simulink model "fm_radio_simulink_v1"  (R2025b)
settings: Solver=VariableStepAuto  StartTime=0.0  StopTime=SimTime  RelTol=1e-3
undefined symbols (not defined in the file): a_de, b_de, decim1, decim2, decim3, decim4, fs_rf
libraries: dspmlti4 x4, dspsrcs4 x1
settings Model: SimulationMode=accelerator  Creator=kmuws  LastModifiedBy=kmuws

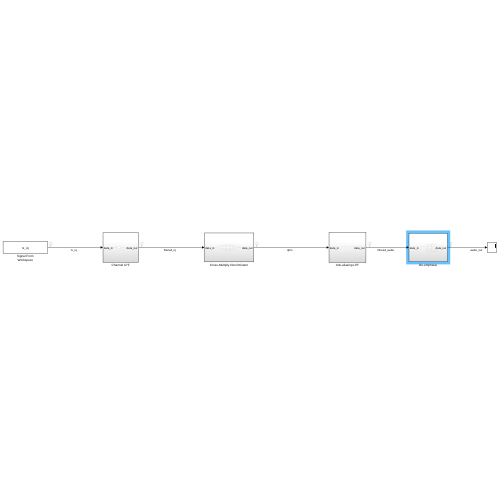
[thumbnail: Simulink's stored preview of the top-level diagram]
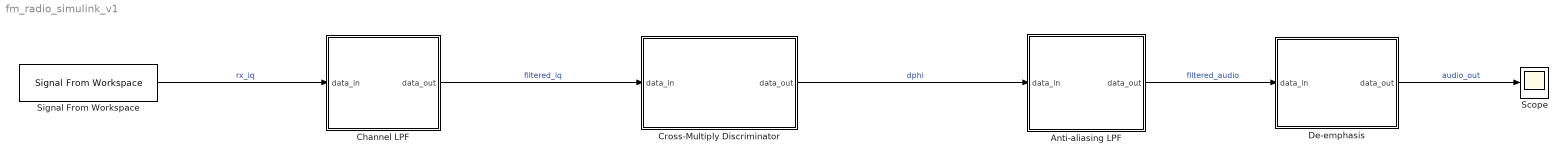
== system fm_radio_simulink_v1 ==
  Anti-aliasing LPF : Subsystem
  Channel LPF : Subsystem
  Cross-Multiply Discriminator : Subsystem
  De-emphasis : Subsystem
  Scope : Scope
      settings: ActiveDisplayYMinimum=-4.7153159237357389  ActiveDisplayYMaximum=3.7645676239050516
  Signal From Workspace : dspsrcs4/Signal From Workspace  X=rx_iq  Ts=1/fs_rf  nsamps=1  OutputAfterFinalValue=Setting to zero  ignoreOrWarnInputAndFrameLengths=off  OutputFrames=off
  wires:
  Signal From Workspace/1 -> Channel LPF/1(data_in)  "rx_iq"
  Channel LPF/1(data_out) -> Cross-Multiply Discriminator/1(data_in)  "filtered_iq"
  Cross-Multiply Discriminator/1(data_out) -> Anti-aliasing LPF/1(data_in)  "dphi"
  Anti-aliasing LPF/1(data_out) -> De-emphasis/1(data_in)  "filtered_audio"
  De-emphasis/1(data_out) -> Scope/1  "audio_out"

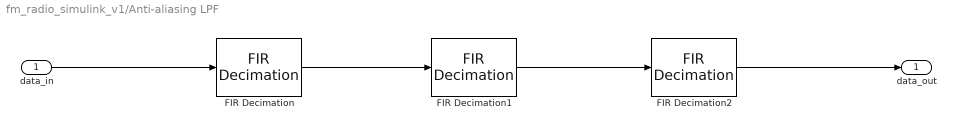
== system fm_radio_simulink_v1/Anti-aliasing LPF ==
  data_in : Inport
  FIR Decimation : dspmlti4/FIR Decimation  FilterSource=Dialog parameters  h=CoefFilter2  D=decim2  filtStruct=Direct form  FilterObject=FDECIM  framing=Enforce single-rate processing  AllowArbitraryInputLength=off  inputOffset=0  outputBufInitCond=0  roundingMode=Floor  overflowMode=off  firstCoeffDataTypeStr=Inherit: Same word length as input  firstCoeffMin=[]  firstCoeffMax=[]  firstCoeffLastDataTypeStr=Inherit: Same word length as input  outputDataTypeStr=Inherit: Same as accumulator  outputMin=[]  outputMax=[]  outputLastDataTypeStr=Inherit: Same as accumulator
  FIR Decimation1 : dspmlti4/FIR Decimation  FilterSource=Dialog parameters  h=CoefFilter3  D=decim3  filtStruct=Direct form  FilterObject=FDECIM  framing=Enforce single-rate processing  AllowArbitraryInputLength=off  inputOffset=0  outputBufInitCond=0  roundingMode=Floor  overflowMode=off  firstCoeffDataTypeStr=Inherit: Same word length as input  firstCoeffMin=[]  firstCoeffMax=[]  firstCoeffLastDataTypeStr=Inherit: Same word length as input  outputDataTypeStr=Inherit: Same as accumulator  outputMin=[]  outputMax=[]  outputLastDataTypeStr=Inherit: Same as accumulator
  FIR Decimation2 : dspmlti4/FIR Decimation  FilterSource=Dialog parameters  h=CoefFilter4  D=decim4  filtStruct=Direct form  FilterObject=FDECIM  framing=Enforce single-rate processing  AllowArbitraryInputLength=off  inputOffset=0  outputBufInitCond=0  roundingMode=Floor  overflowMode=off  firstCoeffDataTypeStr=Inherit: Same word length as input  firstCoeffMin=[]  firstCoeffMax=[]  firstCoeffLastDataTypeStr=Inherit: Same word length as input  outputDataTypeStr=Inherit: Same as accumulator  outputMin=[]  outputMax=[]  outputLastDataTypeStr=Inherit: Same as accumulator
  data_out : Outport
  wires:
  FIR Decimation1/1 -> FIR Decimation2/1
  data_in/1 -> FIR Decimation/1
  FIR Decimation2/1 -> data_out/1
  FIR Decimation/1 -> FIR Decimation1/1

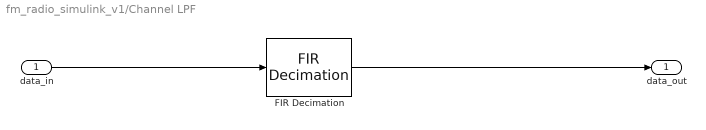
== system fm_radio_simulink_v1/Channel LPF ==
  data_in : Inport
  FIR Decimation : dspmlti4/FIR Decimation  FilterSource=Dialog parameters  h=CoefFilter1  D=decim1  filtStruct=Direct form  FilterObject=FDECIM  framing=Enforce single-rate processing  AllowArbitraryInputLength=off  inputOffset=0  outputBufInitCond=0  roundingMode=Floor  overflowMode=off  firstCoeffDataTypeStr=Inherit: Same word length as input  firstCoeffMin=[]  firstCoeffMax=[]  firstCoeffLastDataTypeStr=Inherit: Same word length as input  outputDataTypeStr=Inherit: Same as accumulator  outputMin=[]  outputMax=[]  outputLastDataTypeStr=Inherit: Same as accumulator
  data_out : Outport
  wires:
  FIR Decimation/1 -> data_out/1
  data_in/1 -> FIR Decimation/1

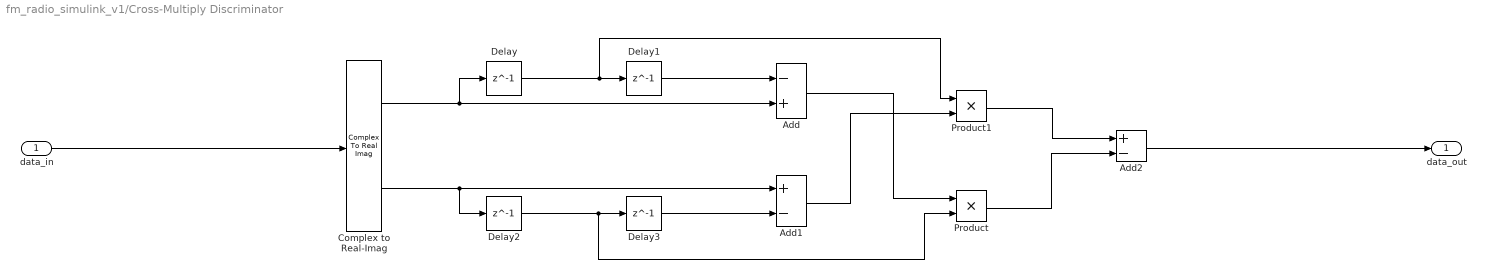
== system fm_radio_simulink_v1/Cross-Multiply Discriminator ==
  data_in : Inport
  Add : Sum  Inputs=-+
  Add1 : Sum  Inputs=+-
  Add2 : Sum  Inputs=+-
  Complex to Real-Imag : ComplexToRealImag
  Delay{,1..3} (4 alike) : Delay  DelayLength=1  InitialCondition=0
  Product : Product
  Product1 : Product
  data_out : Outport
  wires:
  data_in/1 -> Complex to Real-Imag/1
  Product/1 -> Add2/2
  Add1/1 -> Product1/2
  Product1/1 -> Add2/1
  Delay3/1 -> Add1/2
  Delay1/1 -> Add/1
  Complex to Real-Imag/1 -> Add/2, Delay/1
  Add/1 -> Product/1
  Delay/1 -> Delay1/1, Product1/1
  Complex to Real-Imag/2 -> Delay2/1, Add1/1
  Delay2/1 -> Product/2, Delay3/1
  Add2/1 -> data_out/1

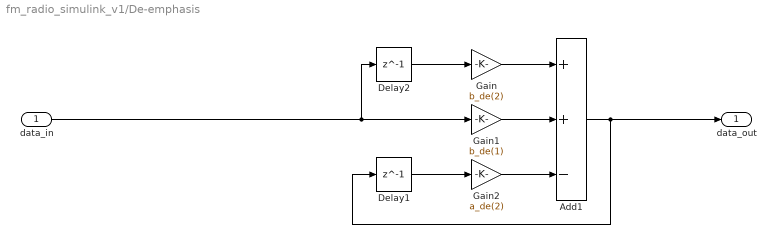
== system fm_radio_simulink_v1/De-emphasis ==
  data_in : Inport
  Add1 : Sum  Inputs=++-
  Delay1 : Delay  DelayLength=1
  Delay2 : Delay  DelayLength=1
  Gain : Gain  Gain=b_de(2)
  Gain1 : Gain  Gain=b_de(1)
  Gain2 : Gain  Gain=a_de(2)
  data_out : Outport
  wires:
  Gain1/1 -> Add1/2
  Delay2/1 -> Gain/1
  Add1/1 -> data_out/1, Delay1/1
  Gain/1 -> Add1/1
  Gain2/1 -> Add1/3
  Delay1/1 -> Gain2/1
  data_in/1 -> Delay2/1, Gain1/1
